simulink model "Week1problem8"  (R2020b)
settings: Solver=VariableStepAuto  StartTime=0.0  StopTime=10.0  RelTol=1e-3
settings Model: Creator=lalit  LastModifiedBy=lalit

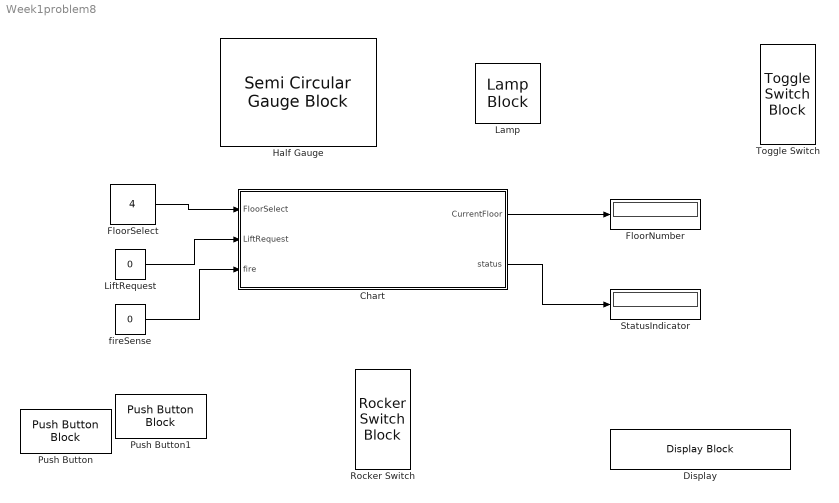
== system Week1problem8 ==
  Chart : Stateflow chart  TreatAsAtomicUnit=on
  Display : DisplayBlock  LabelPosition=Hide  Format=short  Transparency=1
  FloorNumber : Display
  FloorSelect : Constant  Value=4
  Half Gauge : SemiCircularGaugeBlock  ScaleMax=5  TickInterval=1
  Lamp : LampBlock
  LiftRequest : Constant  Value=0
  Push Button : PushButtonBlock
  Push Button1 : PushButtonBlock
  Rocker Switch : RockerSwitchBlock
      settings: Values={{'Off', 'On'}, [0 1]}
  StatusIndicator : Display
  Toggle Switch : ToggleSwitchBlock
      settings: Values={{'Off', 'On'}, [0 1]}
  fireSense : Constant  Value=0
  wires:
  Chart/2(status) -> StatusIndicator/1
  Chart/1(CurrentFloor) -> FloorNumber/1
  fireSense/1 -> Chart/3(fire)
  FloorSelect/1 -> Chart/1(FloorSelect)
  LiftRequest/1 -> Chart/2(LiftRequest)

== stateflow chart Week1problem8/Chart ==
  state LiftOperation [parallel]
    entry:
    status=0;
    settings: executionOrder=2
    state LiftFunctionOn
      (history)
      state GroundFloor
        entry:
        status=1;
        during:
        CurrentFloor=0;
        FloorCheck(CurrentFloor);
        exit:
        status=0;
      state FirstFloor
        entry:
        status=1;
        during:
        CurrentFloor=1;
        FloorCheck(CurrentFloor);
        exit:
        status=0;
      state SecondFloor
        entry:
        status=1;
        during:
        CurrentFloor=2;
        FloorCheck(CurrentFloor);
        exit:
        status=0;
        after(1,sec);
      state ThirdFloor
        entry:
        status=1;
        during:
        CurrentFloor=3;
        FloorCheck(CurrentFloor);
        exit:
        status=0;
        after(1,sec);
      state FourthFloor
        entry:
        status=1
        during:
        CurrentFloor=4;
        FloorCheck(CurrentFloor);
        exit:
        status=0;
      state FifthFloor
        entry:
        status=1;
        during:
        CurrentFloor=5;
        FloorCheck(CurrentFloor);
        exit:
        status=0;
      (default) -> GroundFloor
      GroundFloor -> FirstFloor : up
      FirstFloor -> GroundFloor [order 2] : down
      FirstFloor -> SecondFloor [order 1] : up
      SecondFloor -> FirstFloor [order 2] : down
      SecondFloor -> ThirdFloor [order 1] : up
      ThirdFloor -> SecondFloor [order 2] : down
      ThirdFloor -> FourthFloor [order 1] : up
      FourthFloor -> ThirdFloor [order 1] : down
      FourthFloor -> FifthFloor [order 2] : up
      FifthFloor -> FourthFloor : down
    state LiftFunctionOff
      en:
      status=0;
    (default) -> LiftFunctionOn
    LiftFunctionOff -> LiftFunctionOn : [fire==0]
    LiftFunctionOn -> LiftFunctionOff : [fire==1]
  state Alarm [parallel]
    settings: executionOrder=1
    (default) -> (junction 127) : % Alarm Loop
        | {alarmStatus=fire;}
    (junction 127) -> (junction 129)
    (junction 128) -> (junction 132) [order 2] : [alarmStatus==1]{send(off);}
    (junction 129) -> (junction 128) [order 1] : [1]
    (junction 130) -> (junction 129)
    (junction 128) -> (junction 130) [order 1] : [alarmStatus==0]{send(on);}
    (junction 132) -> (junction 134)
    (junction 129) -> (junction 131) [order 2]
    (junction 134) -> (junction 130)
  state y = FloorCheck(Floor) [function]
    (default) -> (junction 62)
    (junction 62) -> (junction 71) [order 3] : [FloorSelect<Floor]{
        | send(down);
        | disp('LiftMovingDown');}
    (junction 62) -> (junction 65) [order 1] : [FloorSelect>Floor]{
        | send(up);
        | disp('LiftMovingUp');}
    (junction 71) -> (junction 86)
    (junction 62) -> (junction 67) [order 2] : [FloorSelect==Floor]{
        | disp('CurrentFloor');}
    (junction 65) -> (junction 89)
    (junction 86) -> (junction 67)
    (junction 89) -> (junction 67)
    (junction 67) -> (junction 69)
  data: Floor function_input; y function_output; FloorSelect input; LiftRequest input; CurrentFloor output; status output; fire input; alarmStatus local
  events: up local FUNCTION_CALL_EVENT; down local FUNCTION_CALL_EVENT; off local FUNCTION_CALL_EVENT; on local FUNCTION_CALL_EVENT
